simulink model "Boost_MPC"  (R2021a)
settings: Solver=VariableStepAuto  StartTime=0.0  StopTime=inf  RelTol=1e-3
libraries: spsSeriesRLCBranchLib x6, spsVoltageMeasurementLib x4, spsCurrentMeasurementLib x2, spsDCVoltageSourceLib x2, spsDiodeLib x2, spsIGBTLib x2, simulink x1, spspowerguiLib x1
settings Model: Creator=Lenovo  LastModifiedBy=Lenovo

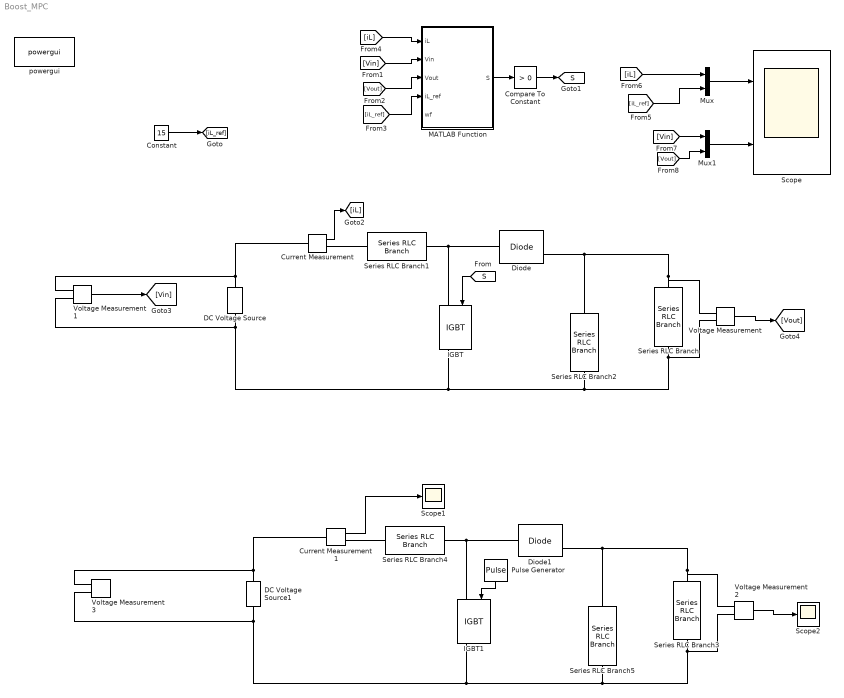
== system Boost_MPC ==
  Compare To Constant : simulink/Logic and Bit Operations/Compare To Constant  relop=>  const=0  OutDataTypeStr=boolean
  Constant : Constant  Value=15
  Current Measurement : spsCurrentMeasurementLib/Current Measurement  PhasorSimulation=off  OutputType=Complex  PSBequivalent=0
  Current Measurement1 : spsCurrentMeasurementLib/Current Measurement  PhasorSimulation=off  OutputType=Complex  PSBequivalent=0
  DC Voltage Source : spsDCVoltageSourceLib/DC Voltage Source  Amplitude=32  Measurements=None
  DC Voltage Source1 : spsDCVoltageSourceLib/DC Voltage Source  Amplitude=32  Measurements=None
  Diode : spsDiodeLib/Diode  Ron=0.001  Lon=0  Vf=0.8  IC=0  UseSnubber=0  Rs=500  Cs=250e-9  Measurements=on
  Diode1 : spsDiodeLib/Diode  Ron=0.001  Lon=0  Vf=0.8  IC=0  UseSnubber=0  Rs=500  Cs=250e-9  Measurements=on
  IGBT : spsIGBTLib/IGBT  Ron=0.001  Lon=0  Vf=1  Tf=1e-6  Tt=2e-6  IC=0  Rs=1e5  Cs=inf  Measurements=on
  IGBT1 : spsIGBTLib/IGBT  Ron=0.001  Lon=0  Vf=1  Tf=1e-6  Tt=2e-6  IC=0  Rs=1e5  Cs=inf  Measurements=on
  MATLAB Function : MATLAB Function  TreatAsAtomicUnit=on
  Mux : Mux  Inputs=2
  Mux1 : Mux  Inputs=2
  Pulse Generator : DiscretePulseGenerator  PulseType=Time based  Period=1/30000  PulseWidth=40
  Scope : Scope  NumInputPorts=2
  Scope1 : Scope
  Scope2 : Scope
  Series RLC Branch : spsSeriesRLCBranchLib/Series RLC Branch  LConnTagsString=__new0  RConnTagsString=__new0  BranchType=R  Resistance=20  Inductance=0  SetiL0=off  InitialCurrent=0  Capacitance=0  Setx0=off  InitialVoltage=0  Measurements=None
  Series RLC Branch1 : spsSeriesRLCBranchLib/Series RLC Branch  LConnTagsString=__new0  RConnTagsString=__new0  BranchType=RL  Resistance=0.2  Inductance=1e-3  SetiL0=off  InitialCurrent=0  Capacitance=1e-6  Setx0=off  InitialVoltage=0  Measurements=None
  Series RLC Branch2 : spsSeriesRLCBranchLib/Series RLC Branch  LConnTagsString=__new0  RConnTagsString=__new0  BranchType=C  Resistance=1  Inductance=1e-3  SetiL0=off  InitialCurrent=0  Capacitance=220e-6  Setx0=off  InitialVoltage=0  Measurements=None
  Series RLC Branch3 : spsSeriesRLCBranchLib/Series RLC Branch  LConnTagsString=__new0  RConnTagsString=__new0  BranchType=R  Resistance=20  Inductance=0  SetiL0=off  InitialCurrent=0  Capacitance=0  Setx0=off  InitialVoltage=0  Measurements=None
  Series RLC Branch4 : spsSeriesRLCBranchLib/Series RLC Branch  LConnTagsString=__new0  RConnTagsString=__new0  BranchType=RL  Resistance=0.2  Inductance=1e-3  SetiL0=off  InitialCurrent=0  Capacitance=1e-6  Setx0=off  InitialVoltage=0  Measurements=None
  Series RLC Branch5 : spsSeriesRLCBranchLib/Series RLC Branch  LConnTagsString=__new0  RConnTagsString=__new0  BranchType=C  Resistance=1  Inductance=1e-3  SetiL0=off  InitialCurrent=0  Capacitance=220e-6  Setx0=off  InitialVoltage=0  Measurements=None
  Voltage Measurement{,1..3} (4 alike) : spsVoltageMeasurementLib/Voltage Measurement  PhasorSimulation=off  OutputType=Complex  PSBequivalent=0
  powergui : spspowerguiLib/powergui  Priority=1  SimulationMode=Discrete  SampleTime=1e-5  frequency=60  Iterations=50  frequencyindice=0  Pbase=100e6  ErrMax=1e-4  UnitsV=kV  UnitsW=MW  buscounter=0  FunctionMessages=off  echomessages=off  EnableUseOfTLC=off  CurrentSourceSwitches=off  DisableSnubberDevices=off  DisableRonSwitches=off  DisableVfSwitches=off  DisplayEquations=off  AutomaticDiscreteSolvers=off  SolverType=Tustin/Backward Euler (TBE)  Interpol=off  ExternalGateDelay=off  methode=off  Ts=100  x0status=blocks  SPID=on  SwTol=0  HookPort=off  NonlinearTolerance=1e-4  nMaxIteration=100  ContinueOnMaxIteration=off  RestoreLinks=warning  ResistiveCurrentMeasurement=off  Frange=[0:2:500]  Ylog=off  Xlog=on  ShowGrid=off  save=off  variable=ZData  structure=0  ZoomFFT=off  StartTime=0.0  cycles=1  DisplayStyle=1  fundamental=60  FreqAxis=off  MaxFrequency=1000  frequencyindicesteady=1  RmsSteady=1  display=off
  tag scope: S=global
  wires:
  [Vin] -> MATLAB Function/2(Vin)
  [Vout] -> MATLAB Function/3(Vout)
  Constant/1 -> [iL_ref]
  [iL_ref] -> MATLAB Function/4(iL_ref)
  [S] -> IGBT/1
  Current Measurement/1 -> [iL]
  [iL] -> MATLAB Function/1(iL)
  Mux/1 -> Scope/1
  Mux1/1 -> Scope/2
  [iL] -> Mux/1
  [iL_ref] -> Mux/2
  [Vin] -> Mux1/1
  [Vout] -> Mux1/2
  MATLAB Function/1(S) -> Compare To Constant/1
  Compare To Constant/1 -> [S]
  Voltage Measurement/1 -> [Vout]
  Voltage Measurement1/1 -> [Vin]
  Voltage Measurement2/1 -> Scope2/1
  Pulse Generator/1 -> IGBT1/1
  Current Measurement1/1 -> Scope1/1
  connections:
  Current Measurement/RConn1 -- Series RLC Branch1/LConn1
  DC Voltage Source/RConn1 -- Voltage Measurement1/LConn1 -- Current Measurement/LConn1
  Voltage Measurement/LConn2 -- Series RLC Branch/RConn1 -- Series RLC Branch2/RConn1 -- IGBT/RConn1 -- Voltage Measurement1/LConn2 -- DC Voltage Source/LConn1
  Diode/LConn1 -- IGBT/LConn1 -- Series RLC Branch1/RConn1
  Series RLC Branch2/LConn1 -- Voltage Measurement/LConn1 -- Series RLC Branch/LConn1 -- Diode/RConn1
  Series RLC Branch5/RConn1 -- Voltage Measurement2/LConn2 -- Series RLC Branch3/RConn1 -- IGBT1/RConn1 -- Voltage Measurement3/LConn2 -- DC Voltage Source1/LConn1
  Diode1/RConn1 -- Series RLC Branch5/LConn1 -- Voltage Measurement2/LConn1 -- Series RLC Branch3/LConn1
  Series RLC Branch4/RConn1 -- Diode1/LConn1 -- IGBT1/LConn1
  DC Voltage Source1/RConn1 -- Voltage Measurement3/LConn1 -- Current Measurement1/LConn1
  Current Measurement1/RConn1 -- Series RLC Branch4/LConn1

== matlab function Boost_MPC/MATLAB Function ==
  data: iL input; S output; Vin input; Vout input; iL_ref input; wf input
function S = MPC_Boost(iL,Vin,Vout,iL_ref,wf)
Ts=10e-6;
L=1e-3;
RL=0.2
States= [1;0];
g_op=1e6;
n_op=1;
persistent S_old;
if isempty(S_old)
    S_old=0;
end

for n=1:2
        iL_k1=(Ts/L)*(Vin-iL*RL-Vout*(1-States(n)))+iL;
        g_sw=abs(States(n)-S_old); 
        g_iL=abs(iL_ref-iL_k1); %cost function
        g = g_iL + g_sw * wf;
        if(g<g_op)
            n_op=n;
            g_op=g;
        end
end 
S=States(n_op);
S_old = S;
